simulink model "stream_data_compatible"  (R2017a)
settings: Solver=VariableStepAuto  StartTime=0.0  StopTime=10.0  RelTol=1e-3
settings Model: Creator=dr446  LastModifiedBy=dr446

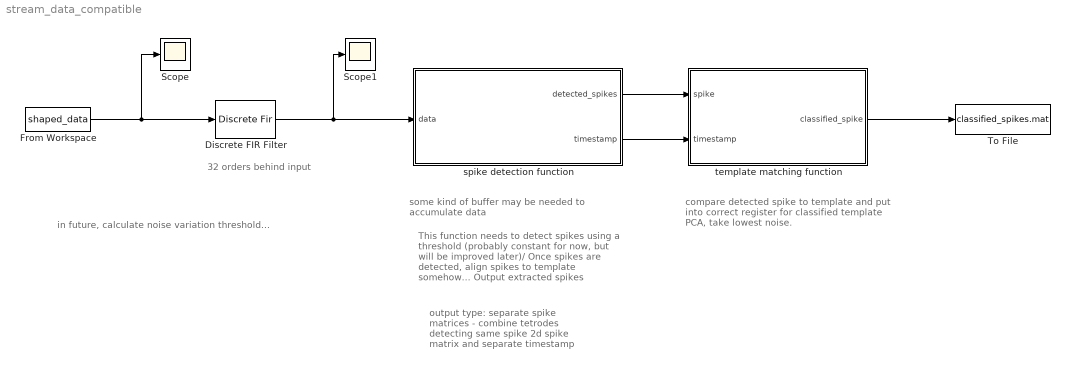
== system stream_data_compatible ==
  note: in future, calculate noise variation threshold...
  note: compare detected spike to template and put into correct register for classified template
      |
      | PCA, take lowest noise.
  note: output type: separate spike matrices - combine tetrodes detecting same spike
      | 2d spike matrix and separate timestamp
  note: 32 orders behind input
  note: This function needs to detect spikes using a threshold (probably constant for now, but will be improved later)/
      | Once spikes are detected, align spikes to template somehow...
      |
      |
      | Output extracted spikes
  note: some kind of buffer may be needed to accumulate data
  Discrete FIR Filter : DiscreteFir  Coefficients="[-0.00256460955632912\t-0.00122763189978458\t0.000415589924103435\t0.000235493840983018\t-0.00460315453054656\t-0.0127730960261749\t-0.0161479251552066\t-0.00701917991322031\t0.00907070223480389\t0.0114671711523351\t-0.0163341202375131\t-0.0606478474288596\t-0.0750999922056139\t-0.0152334366069452\t0.115089684764604\t0.251213077711346\t0.309337809429955\t0.251213077711346\t0.115089684764604\t-0.0152334366069452\t-0.0750999922056139\t-0.0606478474288596\t-0.0163341202375131\t0.0114671711523351\t0.00907070223480389\t-0.00701917991322031\t-0.0161479251552066\t-0.0127730960261749\t-0.00460315453054656\t0.000235493840983018\t0.000415589924103435\t-0.00122763189978458\t-0.00256460955632912]"
  From Workspace : FromWorkspace  VariableName=shaped_data  SampleTime=0
  Scope : Scope
  Scope1 : Scope
  To File : ToFile  Filename=classified_spikes.mat  SaveFormat=Timeseries
  spike detection function : MATLAB Function  TreatAsAtomicUnit=on
  template matching function : MATLAB Function  TreatAsAtomicUnit=on
  wires:
  From Workspace/1 -> Scope/1, Discrete FIR Filter/1
  Discrete FIR Filter/1 -> Scope1/1, spike detection function/1(data)
  spike detection function/1(detected_spikes) -> template matching function/1(spike)
  spike detection function/2(timestamp) -> template matching function/2(timestamp)
  template matching function/1(classified_spike) -> To File/1

== matlab function stream_data_compatible/template matching function ==
  data: spike input; classified_spike output; timestamp input
function classified_spike = template_match(spike, timestamp)

y = u;

== matlab function stream_data_compatible/spike detection function ==
  data: detected_spikes output; data input; timestamp output
% if filtered data is over a certain threshold, take the samples
% immediately to the left and right of the point where the signal crossed
% the threshold.

function [detected_spikes,timestamp] = spike_detect(data) 


isoutlier

y = u;
